simulink model "adrc_controller"  (R2026a)
settings: Solver=FixedStepDiscrete  StartTime=0  StopTime=6  FixedStep=0.004
libraries: simulink x1
settings Model: Creator=Aethor_ca  LastModifiedBy=Aethor_ca
settings DebuggingCC: AlgebraicLoopMsg=error
settings HardwareCC: ProdLargestAtomicInteger=Long  ProdLargestAtomicFloat=Double  ProdHWDeviceType=ARM Compatible->ARM Cortex-M
settings RTWCC: SystemTargetFile=ert.tlc  GenCodeOnly=on  Description=Embedded Coder

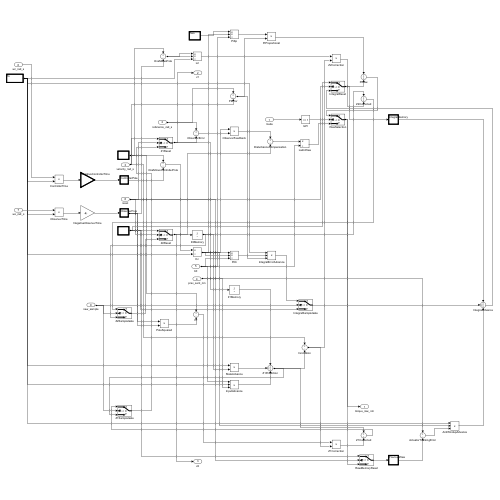
[thumbnail: Simulink's stored preview of the top-level diagram]
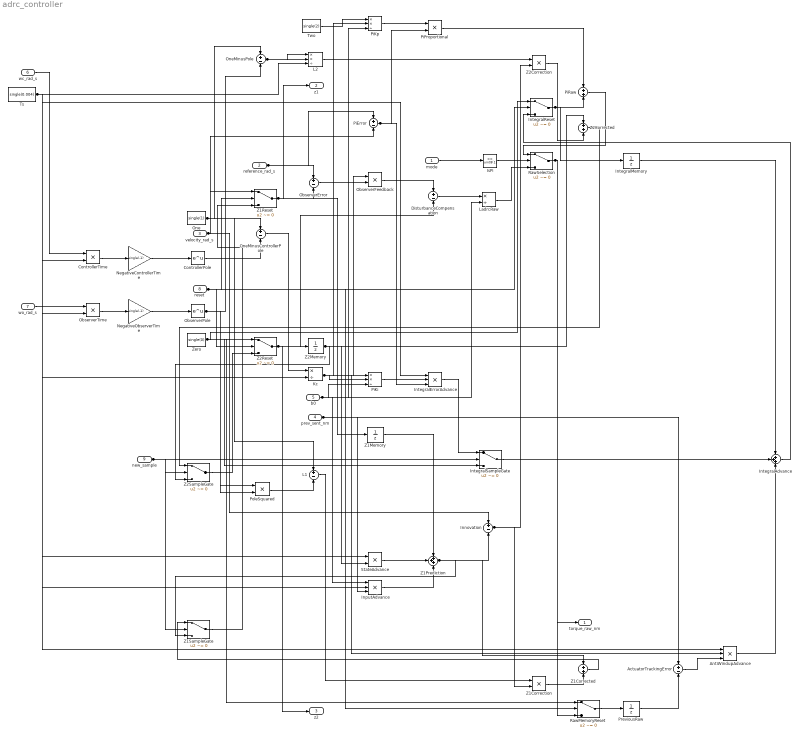
== system adrc_controller ==
  mode : Inport  OutDataTypeStr=uint8  PortDimensions=1  SampleTime=0.004
  reference_rad_s : Inport  Port=2  OutDataTypeStr=single  PortDimensions=1  SampleTime=0.004
  velocity_rad_s : Inport  Port=3  OutDataTypeStr=single  PortDimensions=1  SampleTime=0.004
  prev_sent_nm : Inport  Port=4  OutDataTypeStr=single  PortDimensions=1  SampleTime=0.004
  b0 : Inport  Port=5  OutDataTypeStr=single  PortDimensions=1  SampleTime=0.004
  wc_rad_s : Inport  Port=6  OutDataTypeStr=single  PortDimensions=1  SampleTime=0.004
  wo_rad_s : Inport  Port=7  OutDataTypeStr=single  PortDimensions=1  SampleTime=0.004
  reset : Inport  Port=8  OutDataTypeStr=uint8  PortDimensions=1  SampleTime=0.004
  new_sample : Inport  Port=9  OutDataTypeStr=uint8  PortDimensions=1  SampleTime=0.004
  ActuatorTrackingError : Sum  Inputs=+-  OutDataTypeStr=single
  AntiWindupAdvance : Product  Inputs=***  OutDataTypeStr=single
  ControllerPole : Math
  ControllerTime : Product  Inputs=**  OutDataTypeStr=single
  DisturbanceCompensation : Sum  Inputs=+-  OutDataTypeStr=single
  Innovation : Sum  Inputs=+-  OutDataTypeStr=single
  InputAdvance : Product  Inputs=***  OutDataTypeStr=single
  IntegralAdvance : Sum  Inputs=+++  OutDataTypeStr=single
  IntegralErrorAdvance : Product  Inputs=***  OutDataTypeStr=single
  IntegralMemory : UnitDelay  InitialCondition=single(0)  SampleTime=0.004
  IntegralReset : Switch  Criteria=u2 ~= 0  OutDataTypeStr=single  SaturateOnIntegerOverflow=off  InputSameDT=off
  IntegralSampleGate : Switch  Criteria=u2 ~= 0  OutDataTypeStr=single  SaturateOnIntegerOverflow=off  InputSameDT=off
  IsPi : simulink/Logic and Bit Operations/Compare To Constant  relop===  const=uint8(1)  OutDataTypeStr=boolean
  Kc : Product  Inputs=*/  OutDataTypeStr=single
  L1 : Sum  Inputs=+-  OutDataTypeStr=single
  L2 : Product  Inputs=**/  OutDataTypeStr=single
  LadrcRaw : Product  Inputs=*/  OutDataTypeStr=single
  NegativeControllerTime : Gain  Gain=single(-1)  OutDataTypeStr=single
  NegativeObserverTime : Gain  Gain=single(-1)  OutDataTypeStr=single
  ObserverError : Sum  Inputs=+-  OutDataTypeStr=single
  ObserverFeedback : Product  Inputs=**  OutDataTypeStr=single
  ObserverPole : Math
  ObserverTime : Product  Inputs=**  OutDataTypeStr=single
  One : Constant  Value=single(1)  OutDataTypeStr=single
  OneMinusControllerPole : Sum  Inputs=+-  OutDataTypeStr=single
  OneMinusPole : Sum  Inputs=+-  OutDataTypeStr=single
  PiError : Sum  Inputs=+-  OutDataTypeStr=single
  PiKi : Product  Inputs=**/  OutDataTypeStr=single
  PiKp : Product  Inputs=**/  OutDataTypeStr=single
  PiProportional : Product  Inputs=**  OutDataTypeStr=single
  PiRaw : Sum  OutDataTypeStr=single
  PoleSquared : Product  Inputs=**  OutDataTypeStr=single
  PreviousRaw : UnitDelay  InitialCondition=single(0)  SampleTime=0.004
  RawMemoryReset : Switch  Criteria=u2 ~= 0  OutDataTypeStr=single  SaturateOnIntegerOverflow=off  InputSameDT=off
  RawSelection : Switch  Criteria=u2 ~= 0  OutDataTypeStr=single  SaturateOnIntegerOverflow=off  InputSameDT=off
  StateAdvance : Product  Inputs=**  OutDataTypeStr=single
  Ts : Constant  Value=single(0.004)  OutDataTypeStr=single
  Two : Constant  Value=single(2)  OutDataTypeStr=single
  Z1Corrected : Sum  OutDataTypeStr=single
  Z1Correction : Product  Inputs=**  OutDataTypeStr=single
  Z1Memory : UnitDelay  InitialCondition=single(0)  SampleTime=0.004
  Z1Prediction : Sum  Inputs=+++  OutDataTypeStr=single
  Z1Reset : Switch  Criteria=u2 ~= 0  OutDataTypeStr=single  SaturateOnIntegerOverflow=off  InputSameDT=off
  Z1SampleGate : Switch  Criteria=u2 ~= 0  OutDataTypeStr=single  SaturateOnIntegerOverflow=off  InputSameDT=off
  Z2Corrected : Sum  OutDataTypeStr=single
  Z2Correction : Product  Inputs=**  OutDataTypeStr=single
  Z2Memory : UnitDelay  InitialCondition=single(0)  SampleTime=0.004
  Z2Reset : Switch  Criteria=u2 ~= 0  OutDataTypeStr=single  SaturateOnIntegerOverflow=off  InputSameDT=off
  Z2SampleGate : Switch  Criteria=u2 ~= 0  OutDataTypeStr=single  SaturateOnIntegerOverflow=off  InputSameDT=off
  Zero : Constant  Value=single(0)  OutDataTypeStr=single
  torque_raw_nm : Outport  OutDataTypeStr=single
  z1 : Outport  Port=2  OutDataTypeStr=single
  z2 : Outport  Port=3  OutDataTypeStr=single
  wires:
  Innovation/1 -> Z1Correction/2, Z2Correction/2
  Ts/1 -> InputAdvance/2, StateAdvance/1, IntegralErrorAdvance/1, Kc/2, AntiWindupAdvance/1, ObserverTime/2, L2/3, ControllerTime/2
  reference_rad_s/1 -> PiError/1, ObserverError/1
  wc_rad_s/1 -> ControllerTime/1
  Z1Correction/1 -> Z1Corrected/2
  ObserverTime/1 -> NegativeObserverTime/1
  new_sample/1 -> IntegralSampleGate/2, Z1SampleGate/2, Z2SampleGate/2
  wo_rad_s/1 -> ObserverTime/1
  ControllerTime/1 -> NegativeControllerTime/1
  PiKp/1 -> PiProportional/1
  NegativeControllerTime/1 -> ControllerPole/1
  NegativeObserverTime/1 -> ObserverPole/1
  StateAdvance/1 -> Z1Prediction/2
  Z1SampleGate/1 -> Z1Reset/3
  One/1 -> L1/1, OneMinusPole/1, OneMinusControllerPole/1
  PreviousRaw/1 -> ActuatorTrackingError/2
  ObserverError/1 -> ObserverFeedback/2
  Z2SampleGate/1 -> Z2Reset/3
  velocity_rad_s/1 -> Innovation/1, PiError/2, Z1Reset/1
  ControllerPole/1 -> OneMinusControllerPole/2
  Z2Correction/1 -> Z2Corrected/2
  Zero/1 -> IntegralReset/1, RawMemoryReset/1, IntegralSampleGate/3, Z2Reset/1
  reset/1 -> IntegralReset/2, Z1Reset/2, Z2Reset/2, RawMemoryReset/2
  ObserverPole/1 -> OneMinusPole/2, PoleSquared/1, PoleSquared/2
  ActuatorTrackingError/1 -> AntiWindupAdvance/3
  Z1Corrected/1 -> Z1SampleGate/1
  IsPi/1 -> RawSelection/2
  OneMinusPole/1 -> L2/1, L2/2
  Z1Reset/1 -> Z1Memory/1, z1/1, ObserverError/2
  Two/1 -> PiKp/1
  OneMinusControllerPole/1 -> Kc/1
  LadrcRaw/1 -> RawSelection/3
  mode/1 -> IsPi/1
  prev_sent_nm/1 -> ActuatorTrackingError/1, InputAdvance/3
  Kc/1 -> AntiWindupAdvance/2, PiKp/2, PiKi/2, PiKi/1, ObserverFeedback/1
  Z2Memory/1 -> Z2Corrected/1, StateAdvance/2, Z2SampleGate/3
  Z2Reset/1 -> DisturbanceCompensation/2, Z2Memory/1, z2/1
  PoleSquared/1 -> L1/2
  L2/1 -> Z2Correction/1
  IntegralAdvance/1 -> IntegralReset/3
  b0/1 -> LadrcRaw/2, InputAdvance/1, PiKp/3, PiKi/3
  AntiWindupAdvance/1 -> IntegralAdvance/3
  L1/1 -> Z1Correction/1
  PiRaw/1 -> RawSelection/1
  PiError/1 -> IntegralErrorAdvance/3, PiProportional/2
  ObserverFeedback/1 -> DisturbanceCompensation/1
  PiKi/1 -> IntegralErrorAdvance/2
  Z1Memory/1 -> Z1Prediction/1
  InputAdvance/1 -> Z1Prediction/3
  PiProportional/1 -> PiRaw/1
  DisturbanceCompensation/1 -> LadrcRaw/1
  IntegralErrorAdvance/1 -> IntegralSampleGate/1
  RawMemoryReset/1 -> PreviousRaw/1
  Z1Prediction/1 -> Z1SampleGate/3, Innovation/2, Z1Corrected/1
  IntegralSampleGate/1 -> IntegralAdvance/2
  IntegralReset/1 -> IntegralMemory/1, PiRaw/2
  RawSelection/1 -> torque_raw_nm/1, RawMemoryReset/3
  Z2Corrected/1 -> Z2SampleGate/1
  IntegralMemory/1 -> IntegralAdvance/1
